simulink model "ADPSELSCLTr"  (R2018b)
settings: Solver=ode1  StartTime=0.0  StopTime=20  FixedStep=1/1000  RelTol=1e-3  AbsTol=1e-3  EnableMultiTasking=on
PostLoadFcn:
  | f_Simulink_figureplace
InitFcn:
  | ADPSELSCLTr_PreSim
values from neighbouring files (symbols this model uses):
  basis = 1    [ADPSELSCLTr_PreSim.m]
  beta = 0.1    [ADPSELSCLTr_PreSim.m]
  bias = 0    [ADPSELSCLTr_PreSim.m]
  etaa1 = 0.1    [ADPSELSCLTr_PreSim.m]
  etaa2 = 0.001    [ADPSELSCLTr_PreSim.m]
  etac1 = 1    [ADPSELSCLTr_PreSim.m]
  etac2 = 0    [ADPSELSCLTr_PreSim.m]
  F = 9    [ADPSELSCLTr_PreSim.m]
  fs = 1000    [ADPSELSCLTr_PreSim.m]
  Gamma0 = 1000*eye(L)    [ADPSELSCLTr_PreSim.m]
  GammaBar = 100000    [ADPSELSCLTr_PreSim.m]
  GammaTheta = 1*eye(outlayer)    [ADPSELSCLTr_PreSim.m]
  GSIGMA = zeros(N*L,L)    [ADPSELSCLTr_PreSim.m]
  k = 500    [ADPSELSCLTr_PreSim.m]
  kTheta = M*1    (= 10)    [ADPSELSCLTr_PreSim.m]
  learning = 1    [ADPSELSCLTr_PreSim.m]
  m = 1    [ADPSELSCLTr_PreSim.m]
  M = 10    [ADPSELSCLTr_PreSim.m]
  model = 1    [ADPSELSCLTr_PreSim.m]
  N = length(tc)*length(Ec)^(2)    [ADPSELSCLTr_PreSim.m]
  n = 2    [ADPSELSCLTr_PreSim.m]
  pecutoff = 0.5    [ADPSELSCLTr_PreSim.m]
  projection = 1    [ADPSELSCLTr_PreSim.m]
  Q = [10 0 ; 0 10]    [ADPSELSCLTr_PreSim.m]
  QQ = zeros(N,1)    [ADPSELSCLTr_PreSim.m]
  R = 1    [ADPSELSCLTr_PreSim.m]
  Sidbasis = 15    [ADPSELSCLTr_PreSim.m]
  SIGP = zeros(N*L,2*n)    [ADPSELSCLTr_PreSim.m]
  SIGPF1 = zeros(L,N)    [ADPSELSCLTr_PreSim.m]
  SIGPGD = zeros(N*L,n)    [ADPSELSCLTr_PreSim.m]
  SIGTH = zeros(N*outlayer,N)    [ADPSELSCLTr_PreSim.m]
  SIGTHD = zeros(N*outlayer,N)    [ADPSELSCLTr_PreSim.m]
  theta0 = 0*ones(outlayer,n)    [ADPSELSCLTr_PreSim.m]
  typ = 1    [ADPSELSCLTr_PreSim.m]
  v = 0.005    [ADPSELSCLTr_PreSim.m]
  WaH0 = [0.00981102774694368,1.25468716257868,1.90522222702086,-0.221489942266716,3.96914457427608,-0.434624884727441,0.220704157419489]'    [ADPSELSCLTr_PreSim.m]
  WcH0 = [0.00981102774694368,1.25468716257868,1.90522222702086,-0.221489942266716,3.96914457427608,-0.434624884727441,0.220704157419489]'    [ADPSELSCLTr_PreSim.m]
  x0 = [1; 1]    [ADPSELSCLTr_PreSim.m]
  Ynn = -2.5*(0.5)+2.5*rand(inlayer,p)    [ADPSELSCLTr_PreSim.m]
undefined symbols (not defined in the file or in its folder): g, outlayer
settings Model: Creator=rkamalapurkar  LastModifiedBy=rushik
settings SolverCC: AutoScaleAbsTol=off
settings DataIOCC: SaveFormat=Array  SaveOutput=off  DSMLogging=off  SaveTime=off  SignalLoggingName=ADPTLinearCL
settings OptimizationCC: ExpressionDepthLimit=2147483647  LifeSpan=inf  SimCompilerOptimization=on
settings DebuggingCC: UnderspecifiedInitializationDetection=Classic  MergeDetectMultiDrivingBlocksExec=none  SolverPrmCheckMsg=warning  FcnCallInpInsideContextMsg=warning  StateNameClashWarn=warning  SFUnexpectedBacktrackingDiag=warning  SFNoUnconditionalDefaultTransitionDiag=warning  SFExecutionAtInitializationDiag=none
settings HardwareCC: ProdBitPerPointer=32  ProdBitPerSizeT=32  ProdBitPerPtrDiffT=32  ProdLargestAtomicFloat=None  ProdIntDivRoundTo=Undefined  ProdEndianess=Unspecified  ProdWordSize=32  ProdHWDeviceType=32-bit Generic
settings ModelReferenceCC: PropagateSignalLabelsOutOfModel=off
settings SFSimCC: SimUseLocalCustomCode=off
settings RTWCC: RTWUseLocalCustomCode=off
settings CodeAppCC: StateflowObjectComments=on
settings GRTTargetCC: TargetLangStandard=C89/C90 (ANSI)  GeneratePreprocessorConditionals=Disable all  CombineOutputUpdateFcns=off  GRTInterface=on
settings ConfigComp: CovMetricSettings=dw  CovHtmlReporting=on  CovSaveCumulativeToWorkspaceVar=on  CovSaveSingleToWorkspaceVar=on  CovExternalEMLEnable=off  CovSFcnEnable=off

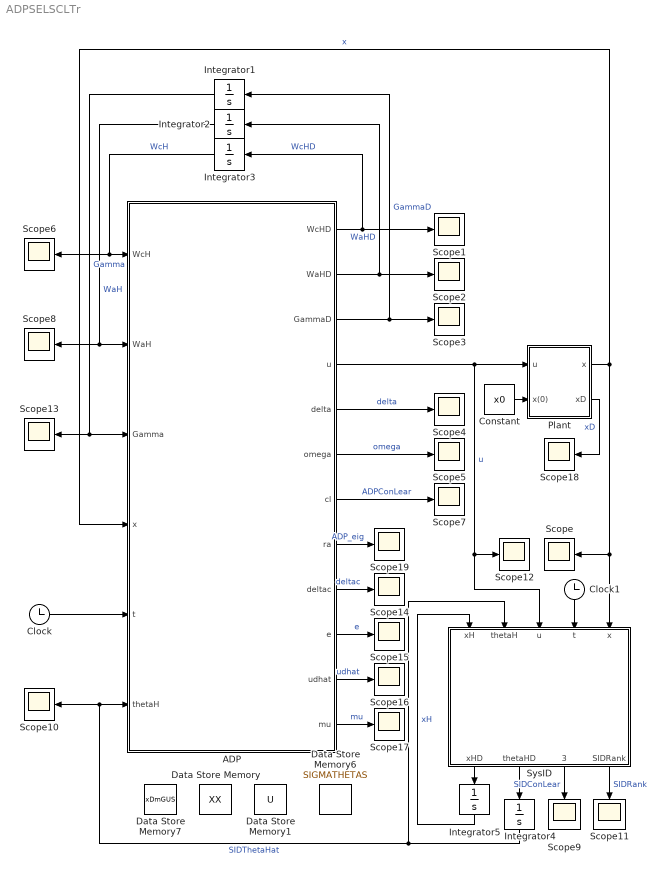
== system ADPSELSCLTr ==
  ADP : MATLAB Function  TreatAsAtomicUnit=on
  Clock : Clock
  Clock1 : Clock
  Constant : Constant  Value=x0
  Data Store Memory : DataStoreMemory  DataStoreName=XX  InitialValue=zeros(n,F)  ShowAdditionalParam=off  OutDataTypeStr=double
  Data Store Memory1 : DataStoreMemory  DataStoreName=U  InitialValue=zeros(m,(F+1)/2)  ShowAdditionalParam=off  OutDataTypeStr=double
  Data Store Memory6 : DataStoreMemory  DataStoreName=SIGMATHETAS  InitialValue=zeros((outlayer),M)  ShowAdditionalParam=off  OutDataTypeStr=double
  Data Store Memory7 : DataStoreMemory  DataStoreName=xDmGUS  InitialValue=zeros(n,M)  ShowAdditionalParam=off  OutDataTypeStr=double
  Integrator1 : Integrator  InitialCondition=Gamma0
  Integrator2 : Integrator  InitialCondition=WaH0
  Integrator3 : Integrator  InitialCondition=WcH0
  Integrator4 : Integrator  InitialCondition=theta0
  Integrator5 : Integrator  InitialCondition=zeros(n,1)
  Plant : Subsystem
  Scope{,1..19} (20 alike) : Scope
  SysID : MATLAB Function  TreatAsAtomicUnit=on
  wires:
  ADP/3(GammaD) -> Integrator1/1, Scope3/1  "GammaD"
  ADP/1(WcHD) -> Integrator3/1, Scope1/1  "WcHD"
  Integrator3/1 -> Scope6/1, ADP/1(WcH)  "WcH"
  ADP/2(WaHD) -> Integrator2/1, Scope2/1  "WaHD"
  Integrator2/1 -> Scope8/1, ADP/2(WaH)  "WaH"
  ADP/5(delta) -> Scope4/1  "delta"
  ADP/6(omega) -> Scope5/1  "omega"
  Integrator1/1 -> Scope13/1, ADP/3(Gamma)  "Gamma"
  Clock/1 -> ADP/5(t)
  ADP/4(u) -> Plant/1(u), SysID/3(u), Scope12/1  "u"
  ADP/7(cl) -> Scope7/1  "ADPConLear"
  Integrator4/1 -> ADP/6(thetaH), Scope10/1, SysID/2(thetaH)  "SIDThetaHat"
  Plant/1(x) -> SysID/5(x), Scope/1, ADP/4(x)  "x"
  Constant/1 -> Plant/2(x(0))
  SysID/1(xHD) -> Integrator5/1
  Integrator5/1 -> SysID/1(xH)  "xH"
  SysID/4(SIDRank) -> Scope11/1  "SIDRank"
  SysID/3(SIDConLear) -> Scope9/1  "SIDConLear"
  SysID/2(thetaHD) -> Integrator4/1
  Clock1/1 -> SysID/4(t)
  ADP/9(deltac) -> Scope14/1  "deltac"
  ADP/10(e) -> Scope15/1  "e"
  ADP/11(udhat) -> Scope16/1  "udhat"
  ADP/12(mu) -> Scope17/1  "mu"
  Plant/2(xD) -> Scope18/1  "xD"
  ADP/8(ra) -> Scope19/1  "ADP_eig"

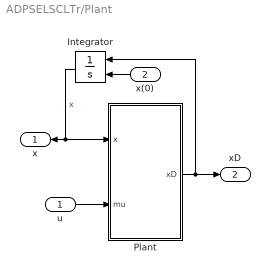
== system ADPSELSCLTr/Plant ==
  u : Inport
  x(0) : Inport  Port=2
  Integrator : Integrator  InitialConditionSource=external  InitialCondition=[1;1;0.0;0.0]
  Plant : MATLAB Function  TreatAsAtomicUnit=on
  x : Outport
  xD : Outport  Port=2
  wires:
  Plant/1(xD) -> Integrator/1, xD/1
  Integrator/1 -> Plant/1(x), x/1  "x"
  u/1 -> Plant/2(mu)
  x(0)/1 -> Integrator/2

== matlab function ADPSELSCLTr/ADP ==
  data: WcH input; WaH input; Gamma input; x input; t input; thetaH input; R parameter; Q parameter; etaa1 parameter; etaa2 parameter; etac1 parameter; v parameter; Ynn parameter; QQ parameter; SIGPF1 parameter; SIGP parameter; SIGPGD parameter; SIGTH parameter; SIGTHD parameter; GSIGMA parameter; model parameter; N parameter; outlayer parameter; typ parameter; WcHD output; WaHD output; GammaD output; u output; delta output; omega output; cl output; ra output; etac2 parameter; beta parameter; GammaBar parameter; projection parameter; deltac output; bias parameter; n parameter; e output; udhat output; mu output; basis parameter; Sidbasis parameter; pecutoff parameter; tf parameter; learning parameter
function [WcHD,WaHD,GammaD,u,delta,omega,cl,ra,deltac,e,udhat,mu]=...
    control(WcH,WaH,Gamma,x,t,thetaH,R,Q,etaa1,etaa2,etac1,v,Ynn,...
    QQ,SIGPF1,SIGP,SIGPGD,SIGTH,SIGTHD,GSIGMA,model,...
    N,outlayer,typ,etac2,beta,GammaBar,projection,bias,n,basis,Sidbasis,...
    pecutoff,tf,learning)
%#codegen
xd = [2*sin(t); 2*cos(t)+2*sin(t)];
% hd = [xd(2)-xd(1); xd(2)-2*xd(1)];
% xd = [2*exp(-t); -2*exp(-0.5*t)];
Ad = [-1 1;-2 1];
hd = Ad*xd;
e = x-xd;
Z = [e;xd];
g=[0; 1];
gplus=[0 1];
gplusd=[0 1];
F1 = [-hd+g*gplusd*hd;hd];
[sigth,~]=ADPSELSCLTr_SIDBasis(x,Sidbasis,bias,Ynn);
[sigthd,~]=ADPSELSCLTr_SIDBasis(xd,Sidbasis,bias,Ynn);
if model==1
    thetaH=[-1 -0.5; 1 -0.5];
end
udhat = gplusd*(hd-thetaH'*sigthd);
G = [g;zeros(size(g))];
[sig_p,L]=ADPSELSCLTr_Basis(Z,basis);         
mu=-0.5*(R\G')*sig_p'*WaH;

pe = -5*sin(5*pi*t) + 10*cos(exp(3)*t);
munew = mu + pe*(t<=tf*pecutoff)*(learning==2);

%% Concurrent Learning

thetaH1 = [thetaH zeros(outlayer,n)];
if typ==1 && learning==1
    GSIGMAWaH = reshape(GSIGMA*WaH,L,N);
%     SIGPTH = 
%     SIGPTH = cell2mat(mat2cell(SIGP*thetaH1',L*ones(N,1),outlayer)');
%     tem=reshape((SIGP*thetaH1')',L,outlayer,N);
%     tem2=reshape(reshape((SIGP*thetaH1')',L,outlayer,N),outlayer,L,N);
%     tem3=permute(reshape(reshape((SIGP*thetaH1')',L,outlayer,N),outlayer,L,N),[2,1,3]);
%     tem4=reshape(tem3,size((SIGP*thetaH1')'));
    SIGPTH=reshape(permute(reshape(reshape((SIGP*thetaH1')',L,outlayer,N),outlayer,L,N),[2,1,3]),L,outlayer*N);
%     reshape(SIGP*thetaH1',L,N*outlayer);
%     SIGPGDTHm = cell2mat(mat2cell(SIGPGD*thetaH',L*ones(N,1),outlayer)');
    SIGPGDTH=reshape(permute(reshape(reshape((SIGPGD*thetaH')',L,outlayer,N),outlayer,L,N),[2,1,3]),L,outlayer*N);
    %reshape(SIGPGD*thetaH',L,N*outlayer);
    if model==0
    Omegac = (SIGPF1 + SIGPTH*SIGTH - SIGPGDTH*SIGTHD - (1/2)*(GSIGMAWaH));
    else
    Omegac = (SIGPF1 - (1/2)*(GSIGMAWaH));
    end
    deltac = Omegac'*WcH+QQ+(1/4)*(GSIGMAWaH'*WaH);
    normm=1./(1.+v.*dot(Omegac.',Omegac.'*Gamma.',2));
    cl = -etac2*Gamma*Omegac*diag(normm)*deltac/N;
    ra=real(min(eig(Omegac*diag(normm)*Omegac')));
else
    deltac=zeros(N,1);
    cl=zeros(size(WcH));
    GSIGMAWaH = zeros(size(WcH,1),N);
    Omegac = zeros(size(WcH,1),N);
    ra=0;
    normm=zeros(N,1);
end

%% ADP
FTH=[thetaH'*sigth-g*gplusd*thetaH'*sigthd;zeros(n,1)];
omega = sig_p*(FTH+F1+G*mu);
Gsigma = sig_p*G*(R\G')*sig_p';
r = e'*Q*e + mu'*R*mu;
delta = WcH'*omega + r;
rho = (1+v*omega'*(Gamma)*omega);
WcHD = (-etac1*Gamma*omega*delta/rho+cl)*(typ==1);
GammaD = (beta*Gamma-Gamma*(omega*omega'/rho^2)*Gamma)*(typ==1)*(norm(Gamma)<=GammaBar);
WaHD = (etaa1*(WcH-WaH)-etaa2*WaH+etac1*Gsigma'*WaH*omega'*WcH/(4*rho)...
    +etac2*GSIGMAWaH*diag(normm)*Omegac'*WcH/(4*N))*(typ==1)*(projection==0)...
    +etaa1*(WcH-WaH)*(typ==1)*(projection==1);
%% Controller
u = munew+udhat;

== matlab function ADPSELSCLTr/Plant/Plant ==
  data: xD output; x input; mu input
function xD = dynamics(x,mu)
%#codegen
A=[-1 1; -0.5 -0.5];
F=A*x;
G=[0; 1];
xD = F+G*mu;

== matlab function ADPSELSCLTr/SysID ==
  settings: updateMethod=DISCRETE
  data: xH input; xHD output; thetaH input; thetaHD output; u input; SIDConLear output; SIDRank output; t input; x input; k parameter; GammaTheta parameter; kTheta parameter; M parameter; XX data_store_memory; fs parameter; F parameter; g parameter; U data_store_memory; typ parameter; model parameter; Ynn parameter; bias parameter; SIGMATHETAS data_store_memory; xDmGUS data_store_memory; Sidbasis parameter
function [xHD,thetaHD,SIDConLear,SIDRank] = Control(xH,thetaH,u,t,x,k,...
    GammaTheta,kTheta,M,fs,F,g,typ,model,Ynn,bias,Sidbasis)
%#codegen
% This simulink block implements concurrent-learning based system
% identification using a Savitzky–Golay smoothing filter for state
% derivative computation. 
% fs: Sampling frequency
% M: number of stored data points
% F: Savitzky–Golay filter window length
% g: Savitzky–Golay filter differentiation matrix

global XX; % Data store memory for storing the values of x
global U; % Data store memory for storing the values of u
global SIGMATHETAS; % Data store for storing the values of sigth,
           % made of sigth matrices stacked in a row
global xDmGUS; % Data store memory for storing the values of xDot-G*u

%Dynamics
G=[0; 1];

if typ == 1 && model~=1
ite=round(t*fs)+1; % Current iteration number
xT = x-xH;

% Basis functions
[sigth,~]=ADPSELSCLTr_SIDBasis(x,Sidbasis,bias,Ynn);

% At every time ite store the past F values of the state. Note that 
% Q*g(:,2)/(1/fs) gives the state derivative at ite-(F-1)/2
if ite<=F
    XX(:,ite)=x;
else
    XX = [XX(:,2:F) x];
end

% At every time ite store the past (F+1)/2 values of the control. Actually, 
% we only need the value of u at ite-(F-1)/2. However, I could not find a 
% way to store just that single value. Also, even if U is initialized as a 
% row vector, MATLAB seems to think its a column.
if ite<=(F+1)/2
    U(ite)=u;
else
    U = [U(2:(F+1)/2); u];
end

% The state derivative information is only available if ite>=F use
% singular value maximization algorithm to replace elements of SIGMATHETAS
% and XDmGUS with new data. At each time ite, the value of the 
% state at ite-(F-1)/2 can be found in XX(:,(F+1)/2)
index=0;
if ite>=F
    xj=XX(:,(F+1)/2);
    [sigthj,~]=ADPSELSCLTr_SIDBasis(xj,Sidbasis,bias,Ynn);
    REGste1 = SIGMATHETAS*SIGMATHETAS'; % Compute Summation
    svd1=min(svd(REGste1));
    for i=1:M
         % Store existing data in a temporary variable
        SIGMATHETASte=SIGMATHETAS;
        % Replac i'th sigth matrix with sigthj
        SIGMATHETASte(:,i)=sigthj;
        REGste2 = SIGMATHETASte*SIGMATHETASte'; % Compute Summation
        svd2=min(svd(REGste2)); % Minimum singular value after replacement
        if svd1<svd2 % If replacement results in a higher singular value,
            index=i; % note the index of replacement and
            svd1=svd2; % keep searching for an even higher singular value.           
        end
    end
    
% At this point, index points to the matrix sigth in the stack 
% SIGMATHETAS which, when replaced with the new matrix sigthj,
% results in the highest singular value.
% If index=0, the new data point is discarded. Otherwise, the stack
% SIGMATHETAS, and correspondingly the stack xDmGUS is updated with the 
% new data point.
% Note that since there is a delay of (F-1)/2 for derivative computation,
% the "new" data point we are talking about is the one that was recorded 
% (F-1)/2 steps ago.
    if index ~= 0
        SIGMATHETAS(:,index)=sigthj;
        uj=U(1,1);
        xDj=XX*g(:,2)/(1/fs);
        Gj = [0; 1]; 
        xDmGUS(:,index)=xDj-Gj*uj;
    end
end

xHD = thetaH'*sigth + G*u + k*xT;

% Final computation for the concurrent learning-based component of the
% adaptive update law. The concurrent learning component is zero for the
% first F timesteps.
REGs = SIGMATHETAS*SIGMATHETAS'*(ite>=F);
SIDRank = min(svd(REGs)); % For plots
REG1s = SIGMATHETAS*xDmGUS'*(ite>=F);
SIDConLear = (REG1s-REGs*thetaH)/M;
thetaHD = (GammaTheta*sigth*xT' + kTheta*GammaTheta*SIDConLear);
else
SIDConLear = zeros(size(thetaH));
SIDRank = 0;
xHD = zeros(size(xH));    
thetaHD = zeros(size(thetaH));
end
